simulink model "smc_4"  (R2017a)
settings: Solver=VariableStepAuto  StartTime=0.0  StopTime=10  RelTol=1e-3
undefined symbols (not defined in the file): A, Asys, Bsys, c, Csys, Dsys, k, sin_input, w
settings Model: Creator=Matteo  LastModifiedBy=Matteo

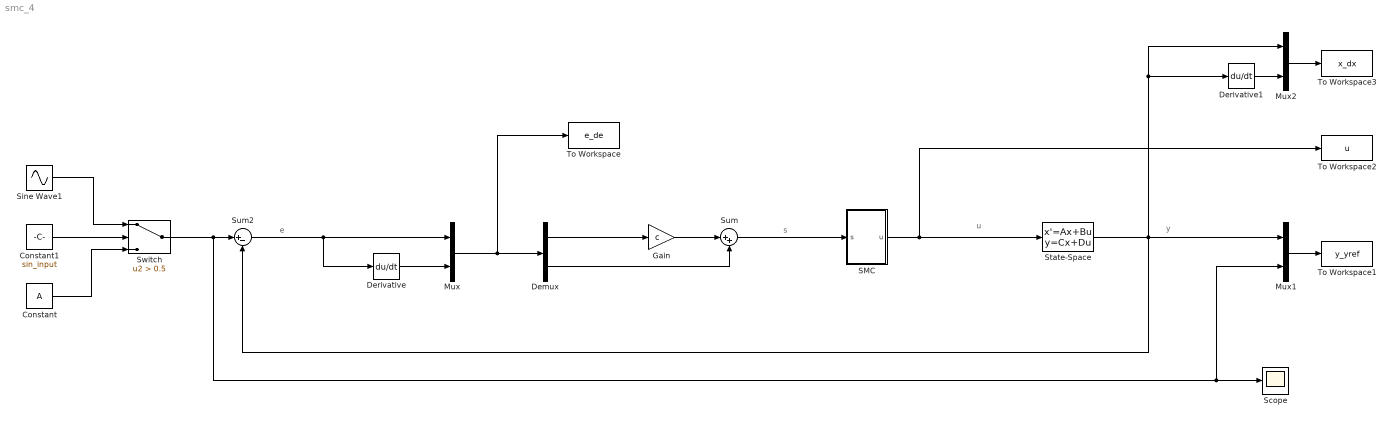
== system smc_4 ==
  note: y
  note: s
  note: e
  note: u
  Constant : Constant  Value=A
  Constant1 : Constant  Value=sin_input
  Demux : Demux  Outputs=2
  Derivative : Derivative
  Derivative1 : Derivative
  Gain : Gain  Gain=c
  Mux : Mux  Inputs=2
  Mux1 : Mux  Inputs=2
  Mux2 : Mux  Inputs=2
  SMC : Subsystem
  Scope : Scope
  Sine Wave1 : Sin  Amplitude=A  Frequency=w  SampleTime=0
  State-Space : StateSpace  A=Asys  B=Bsys  C=Csys  D=Dsys  X0=0
  Sum : Sum  Inputs=|++
  Sum2 : Sum  Inputs=|+-
  Switch : Switch  Criteria=u2 > Threshold  Threshold=0.5
  To Workspace : ToWorkspace  VariableName=e_de  SampleTime=-1
  To Workspace1 : ToWorkspace  VariableName=y_yref  SaveFormat=Structure With Time  SampleTime=-1
  To Workspace2 : ToWorkspace  VariableName=u  SaveFormat=Structure With Time  SampleTime=-1
  To Workspace3 : ToWorkspace  VariableName=x_dx  SampleTime=-1
  wires:
  Gain/1 -> Sum/1
  SMC/1(u) -> State-Space/1, To Workspace2/1
  Demux/2 -> Sum/2
  Derivative/1 -> Mux/2
  Sum/1 -> SMC/1(s)
  Sum2/1 -> Derivative/1, Mux/1
  State-Space/1 -> Derivative1/1, Mux2/1, Sum2/2, Mux1/1
  Mux/1 -> To Workspace/1, Demux/1
  Mux2/1 -> To Workspace3/1
  Switch/1 -> Mux1/2, Scope/1, Sum2/1
  Mux1/1 -> To Workspace1/1
  Demux/1 -> Gain/1
  Derivative1/1 -> Mux2/2
  Constant1/1 -> Switch/2
  Sine Wave1/1 -> Switch/1
  Constant/1 -> Switch/3

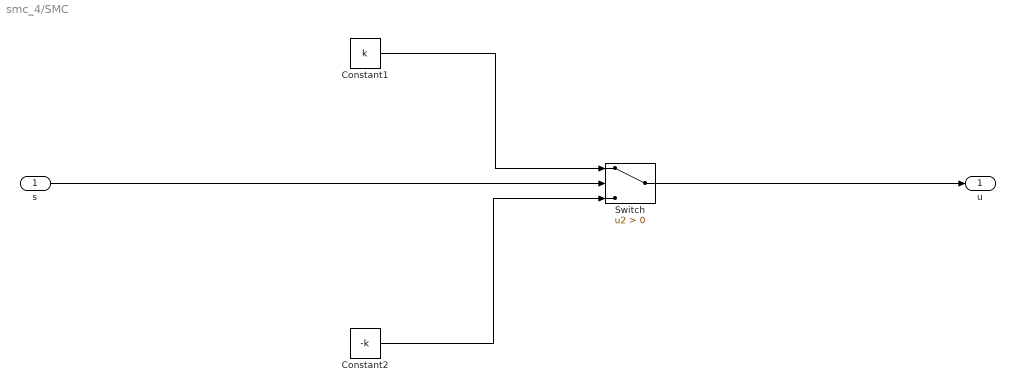
== system smc_4/SMC ==
  s : Inport
  Constant1 : Constant  Value=k
  Constant2 : Constant  Value=-k
  Switch : Switch  Criteria=u2 > Threshold  ZeroCross=off
  u : Outport
  wires:
  Constant1/1 -> Switch/1
  Constant2/1 -> Switch/3
  Switch/1 -> u/1
  s/1 -> Switch/2
